simulink model "Comm_vec1111"  (R2018b)
settings: Solver=VariableStepAuto  StartTime=0.0  StopTime=4  MaxStep=1/(100*fn)  RelTol=1e-3
values from neighbouring files (symbols this model uses):
  A = sqrt(2/3)*[1 -0.5 -0.5; 0 sqrt(3)/2 -sqrt(3)/2; sqrt(0.5) sqrt(0.5) sqrt(0.5)]    [Comm_Vect.m]    (also in clarke_conc.m)
  Ai = inv(A)    [Comm_Vect.m]    (also in clarke_conc.m)
  fv = 0.0033    [Comm_Vect.m]    (also in clarke_conc.m)
  J = 0.05    [Comm_Vect.m]    (also in clarke_conc.m)
  Kond = 178    [Comm_Vect.m]
  Kpd = Rs/Kond    (= 0.0589887640449)    [Comm_Vect.m]
  Kpq = Rs/Kond    (= 0.0589887640449)    [Comm_Vect.m]
  Kpv = 1/Kond    (= 0.00561797752809)    [Comm_Vect.m]
  Ld = 0.245    [Comm_Vect.m]    (also in clarke_conc.m)
  Lq = 0.245    [Comm_Vect.m]    (also in clarke_conc.m)
  p = 60*fn/Nn    (= 2)    [Comm_Vect.m]    (also in clarke_conc.m)
  phi_f = 0.711    [Comm_Vect.m]    (also in clarke_conc.m)
  Rs = 10.5    [Comm_Vect.m]    (also in clarke_conc.m)
  Tid = Ld/Rs    (= 0.0233333333333)    [Comm_Vect.m]
  Tiq = Lq/Rs    (= 0.0233333333333)    [Comm_Vect.m]
  Tiv = J/fv    (= 15.1515151515)    [Comm_Vect.m]
  ws = 2*pi*fn/p    (= 157.079632679)    [Comm_Vect.m]    (also in clarke_conc.m)
undefined symbols (not defined in the file or in its folder): jsin
settings Model: Creator=cindyiskandar  LastModifiedBy=cindyiskandar

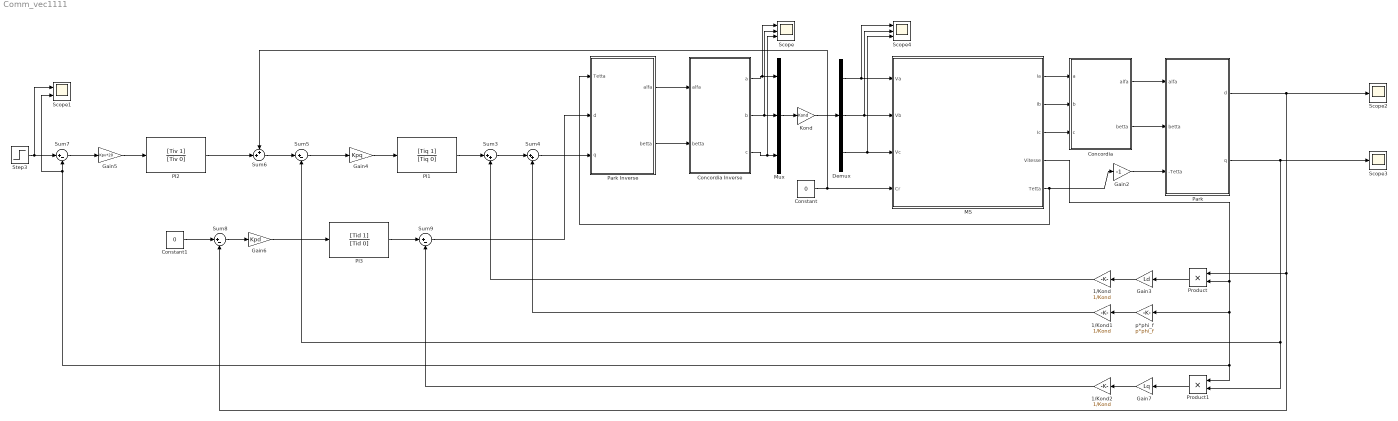
== system Comm_vec1111 ==
  1/Kond : Gain  Gain=1/Kond
  1/Kond1 : Gain  Gain=1/Kond
  1/Kond2 : Gain  Gain=1/Kond
  "Concordia " : Subsystem
  "Concordia Inverse " : Subsystem
  Constant : Constant  Value=0
  Constant1 : Constant  Value=0
  Demux : Demux  Outputs=3
  Gain2 : Gain  Gain=-1
  Gain3 : Gain  Gain=Ld
  Gain4 : Gain  Gain=Kpq
  Gain5 : Gain  Gain=Kpv*20
  Gain6 : Gain  Gain=Kpd
  Gain7 : Gain  Gain=Lq
  Kond : Gain  Gain=Kond
  MS : Subsystem
  Mux : Mux  Inputs=3
  PI1 : TransferFcn  Numerator=[Tiq 1]  Denominator=[Tiq 0]
  PI2 : TransferFcn  Numerator=[Tiv 1]  Denominator=[Tiv 0]
  PI3 : TransferFcn  Numerator=[Tid 1]  Denominator=[Tid 0]
  Park : Subsystem
  Park Inverse : Subsystem
  Product : Product
  Product1 : Product
  Scope : Scope  NumInputPorts=3
  Scope1 : Scope  NumInputPorts=2
  Scope2 : Scope
  Scope3 : Scope
  Scope4 : Scope  NumInputPorts=3
  Step3 : Step  Time=0  After=ws  SampleTime=0
  Sum3 : Sum  Inputs=|++
  Sum4 : Sum  Inputs=|++
  Sum{5,7..9} (4 alike) : Sum  Inputs=|+-
  Sum6 : Sum  Inputs=++|
  "p*phi_f " : Gain  Gain=p*phi_f
  wires:
  Park Inverse/2(betta) -> "Concordia Inverse "/2(betta)
  Step3/1 -> Scope1/1, Sum7/1
  "Concordia "/2("betta ") -> Park/2("betta ")
  Sum3/1 -> Sum4/1
  1/Kond2/1 -> Sum9/2
  "p*phi_f "/1 -> 1/Kond1/1
  Product/1 -> Gain3/1
  Gain5/1 -> PI2/1
  Constant1/1 -> Sum8/1
  Park/1(d) -> Scope2/1, Product/1, Sum8/2
  "Concordia Inverse "/2(b) -> Scope/2, Mux/2
  1/Kond1/1 -> Sum4/2
  PI1/1 -> Sum3/1
  Product1/1 -> Gain7/1
  Sum7/1 -> Gain5/1
  MS/5("Tetta ") -> Gain2/1, Park Inverse/1("Tetta ")
  Sum8/1 -> Gain6/1
  Park Inverse/1(alfa) -> "Concordia Inverse "/1(alfa)
  Gain7/1 -> 1/Kond2/1
  Mux/1 -> Kond/1
  "Concordia Inverse "/1(a) -> Scope/1, Mux/1
  Gain2/1 -> Park/3(-Tetta)
  MS/4(Vitesse) -> "p*phi_f "/1, Product1/1, Scope1/2, Sum7/2, Product/2
  Sum5/1 -> Gain4/1
  MS/3(Ic) -> "Concordia "/3(c)
  MS/2(Ib) -> "Concordia "/2("b ")
  Sum9/1 -> Park Inverse/2(d)
  Gain3/1 -> 1/Kond/1
  Gain6/1 -> PI3/1
  1/Kond/1 -> Sum3/2
  "Concordia "/1(alfa) -> Park/1(alfa)
  Gain4/1 -> PI1/1
  PI3/1 -> Sum9/1
  MS/1(Ia) -> "Concordia "/1("a ")
  Constant/1 -> MS/4(Cr), Sum6/1
  PI2/1 -> Sum6/2
  Sum4/1 -> Park Inverse/3("q ")
  Kond/1 -> Demux/1
  Park/2(q) -> Scope3/1, Product1/2, Sum5/2
  "Concordia Inverse "/3(c) -> Scope/3, Mux/3
  Demux/3 -> Scope4/3, MS/3(Vc)
  Demux/1 -> Scope4/1, MS/1(Va)
  Demux/2 -> MS/2(Vb), Scope4/2
  Sum6/1 -> Sum5/1

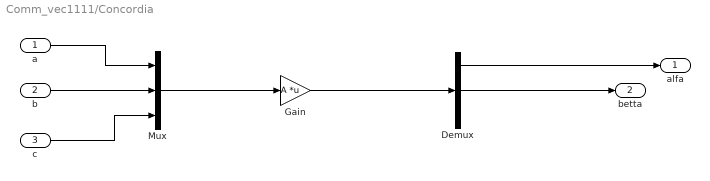
== system Comm_vec1111/Concordia  ==
  "a " : Inport
  "b " : Inport  Port=2
  c : Inport  Port=3
  Demux : Demux  Outputs=3
  Gain : Gain  Gain=A  Multiplication=Matrix(K*u) (u vector)
  Mux : Mux  Inputs=3
  alfa : Outport
  "betta " : Outport  Port=2
  wires:
  Demux/1 -> alfa/1
  "a "/1 -> Mux/1
  Mux/1 -> Gain/1
  Gain/1 -> Demux/1
  "b "/1 -> Mux/2
  c/1 -> Mux/3
  Demux/2 -> "betta "/1

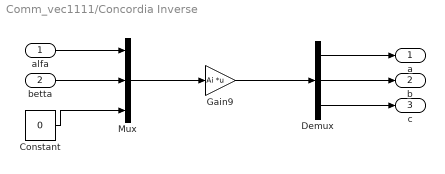
== system Comm_vec1111/Concordia Inverse  ==
  alfa : Inport
  betta : Inport  Port=2
  Constant : Constant  Value=0
  Demux : Demux  Outputs=3
  Gain9 : Gain  Gain=Ai  Multiplication=Matrix(K*u) (u vector)
  Mux : Mux  Inputs=3
  a : Outport
  b : Outport  Port=2
  c : Outport  Port=3
  wires:
  Demux/3 -> c/1
  Gain9/1 -> Demux/1
  Demux/1 -> a/1
  Demux/2 -> b/1
  betta/1 -> Mux/2
  alfa/1 -> Mux/1
  Mux/1 -> Gain9/1
  Constant/1 -> Mux/3

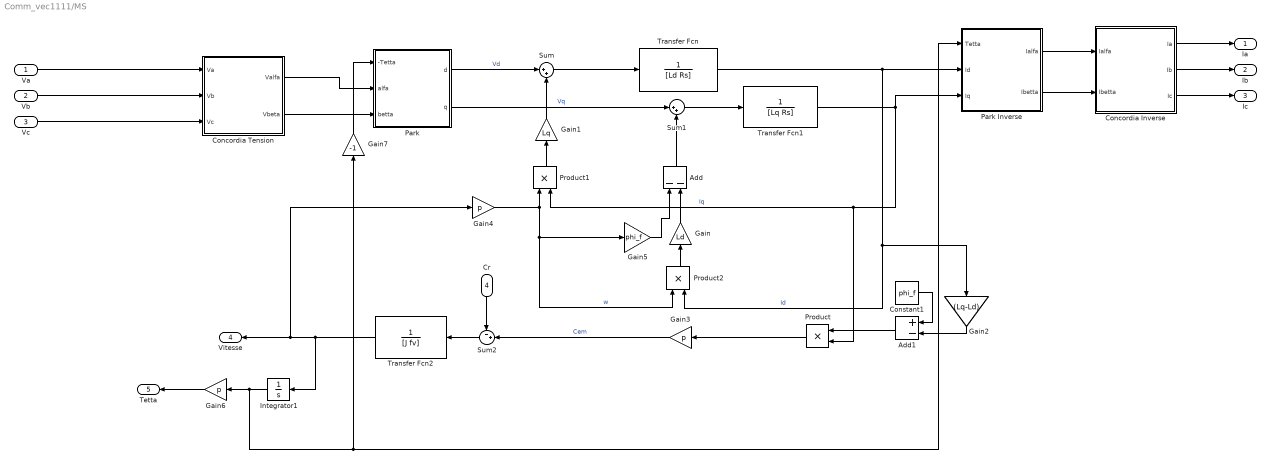
== system Comm_vec1111/MS ==
  Va : Inport
  Vb : Inport  Port=2
  Vc : Inport  Port=3
  Cr : Inport  Port=4
  Add : Sum  Inputs=--
  Add1 : Sum  Inputs=+-
  "Concordia Tension " : Subsystem
  "Concordia Inverse " : Subsystem
  Constant1 : Constant  Value=phi_f
  Gain : Gain  Gain=Ld
  Gain1 : Gain  Gain=Lq
  Gain2 : Gain  Gain=(Lq-Ld)
  Gain3 : Gain  Gain=p
  Gain4 : Gain  Gain=p
  Gain5 : Gain  Gain=phi_f
  Gain6 : Gain  Gain=p
  Gain7 : Gain  Gain=-1
  Integrator1 : Integrator  InitialCondition=ws
  Park : Subsystem
  Park Inverse : Subsystem
  Product : Product
  Product1 : Product
  Product2 : Product
  Sum : Sum  Inputs=|++
  Sum1 : Sum  Inputs=|++
  Sum2 : Sum  Inputs=-+|
  Transfer Fcn : TransferFcn  Denominator=[Ld Rs]
  Transfer Fcn1 : TransferFcn  Denominator=[Lq Rs]
  Transfer Fcn2 : TransferFcn  Denominator=[J fv]
  Ia : Outport
  Ib : Outport  Port=2
  Ic : Outport  Port=3
  Vitesse : Outport  Port=4
  "Tetta " : Outport  Port=5
  wires:
  Gain2/1 -> Add1/2
  Sum1/1 -> Transfer Fcn1/1
  Gain1/1 -> Sum/2
  Va/1 -> "Concordia Tension "/1("Va ")
  Gain/1 -> Add/2
  "Concordia Inverse "/2(Ib) -> Ib/1
  Vb/1 -> "Concordia Tension "/2("Vb ")
  Constant1/1 -> Add1/1
  Transfer Fcn1/1 -> Park Inverse/3("Iq "), Product1/2, Product/2  "Iq"
  "Concordia Inverse "/3(Ic) -> Ic/1
  Add1/1 -> Product/1
  Add/1 -> Sum1/2
  Park Inverse/2(Ibetta) -> "Concordia Inverse "/2(Ibetta)
  Park Inverse/1(Ialfa) -> "Concordia Inverse "/1(Ialfa)
  Sum/1 -> Transfer Fcn/1
  "Concordia Tension "/2("Vbeta ") -> Park/3("betta ")
  "Concordia Tension "/1(Valfa) -> Park/2(alfa)
  Vc/1 -> "Concordia Tension "/3(Vc)
  "Concordia Inverse "/1(Ia) -> Ia/1
  Park/1(d) -> Sum/1  "Vd"
  Transfer Fcn/1 -> Product2/2, Gain2/1, Park Inverse/2(Id)  "Id"
  Park/2(q) -> Sum1/1  "Vq"
  Product/1 -> Gain3/1
  Cr/1 -> Sum2/1
  Sum2/1 -> Transfer Fcn2/1
  Transfer Fcn2/1 -> Gain4/1, Vitesse/1, Integrator1/1
  Product1/1 -> Gain1/1
  Gain4/1 -> Product2/1, Gain5/1, Product1/1  "w"
  Product2/1 -> Gain/1
  Gain5/1 -> Add/1
  Gain6/1 -> "Tetta "/1
  Integrator1/1 -> Gain7/1, Park Inverse/1("Tetta "), Gain6/1
  Gain7/1 -> Park/1(-Tetta)
  Gain3/1 -> Sum2/2  "Cem"

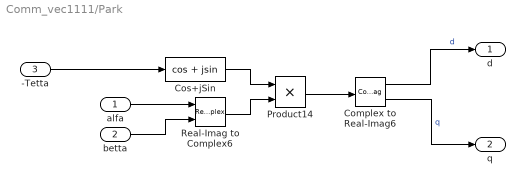
== system Comm_vec1111/Park ==
  alfa : Inport
  "betta " : Inport  Port=2
  -Tetta : Inport  Port=3
  Complex to Real-Imag6 : ComplexToRealImag
  Cos+jSin : Trigonometry  Operator=cos + jsin
  Product14 : Product
  Real-Imag to Complex6 : RealImagToComplex
  d : Outport
  q : Outport  Port=2
  wires:
  alfa/1 -> Real-Imag to Complex6/1
  Product14/1 -> Complex to Real-Imag6/1
  "betta "/1 -> Real-Imag to Complex6/2
  Complex to Real-Imag6/1 -> d/1  "d"
  Complex to Real-Imag6/2 -> q/1  "q"
  Real-Imag to Complex6/1 -> Product14/2
  Cos+jSin/1 -> Product14/1
  -Tetta/1 -> Cos+jSin/1

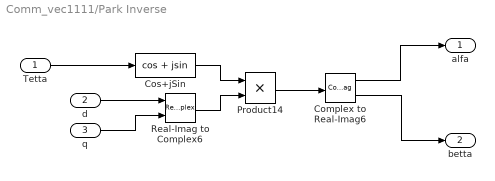
== system Comm_vec1111/Park Inverse ==
  "Tetta " : Inport
  d : Inport  Port=2
  "q " : Inport  Port=3
  Complex to Real-Imag6 : ComplexToRealImag
  Cos+jSin : Trigonometry  Operator=cos + jsin
  Product14 : Product
  Real-Imag to Complex6 : RealImagToComplex
  alfa : Outport
  betta : Outport  Port=2
  wires:
  d/1 -> Real-Imag to Complex6/1
  Product14/1 -> Complex to Real-Imag6/1
  "q "/1 -> Real-Imag to Complex6/2
  Complex to Real-Imag6/1 -> alfa/1
  Complex to Real-Imag6/2 -> betta/1
  Real-Imag to Complex6/1 -> Product14/2
  Cos+jSin/1 -> Product14/1
  "Tetta "/1 -> Cos+jSin/1

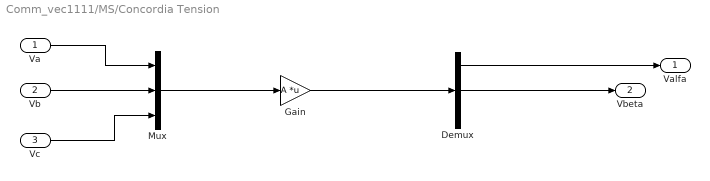
== system Comm_vec1111/MS/Concordia Tension  ==
  "Va " : Inport
  "Vb " : Inport  Port=2
  Vc : Inport  Port=3
  Demux : Demux  Outputs=3
  Gain : Gain  Gain=A  Multiplication=Matrix(K*u) (u vector)
  Mux : Mux  Inputs=3
  Valfa : Outport
  "Vbeta " : Outport  Port=2
  wires:
  Demux/1 -> Valfa/1
  "Va "/1 -> Mux/1
  Mux/1 -> Gain/1
  Gain/1 -> Demux/1
  "Vb "/1 -> Mux/2
  Vc/1 -> Mux/3
  Demux/2 -> "Vbeta "/1

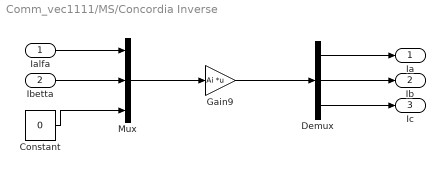
== system Comm_vec1111/MS/Concordia Inverse  ==
  Ialfa : Inport
  Ibetta : Inport  Port=2
  Constant : Constant  Value=0
  Demux : Demux  Outputs=3
  Gain9 : Gain  Gain=Ai  Multiplication=Matrix(K*u) (u vector)
  Mux : Mux  Inputs=3
  Ia : Outport
  Ib : Outport  Port=2
  Ic : Outport  Port=3
  wires:
  Demux/3 -> Ic/1
  Gain9/1 -> Demux/1
  Demux/1 -> Ia/1
  Demux/2 -> Ib/1
  Ibetta/1 -> Mux/2
  Ialfa/1 -> Mux/1
  Mux/1 -> Gain9/1
  Constant/1 -> Mux/3

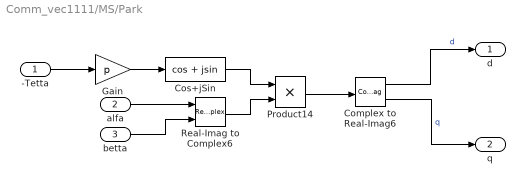
== system Comm_vec1111/MS/Park ==
  -Tetta : Inport
  alfa : Inport  Port=2
  "betta " : Inport  Port=3
  Complex to Real-Imag6 : ComplexToRealImag
  Cos+jSin : Trigonometry  Operator=cos + jsin
  Gain : Gain  Gain=p
  Product14 : Product
  Real-Imag to Complex6 : RealImagToComplex
  d : Outport
  q : Outport  Port=2
  wires:
  alfa/1 -> Real-Imag to Complex6/1
  Product14/1 -> Complex to Real-Imag6/1
  "betta "/1 -> Real-Imag to Complex6/2
  Complex to Real-Imag6/1 -> d/1  "d"
  Complex to Real-Imag6/2 -> q/1  "q"
  Real-Imag to Complex6/1 -> Product14/2
  Cos+jSin/1 -> Product14/1
  Gain/1 -> Cos+jSin/1
  -Tetta/1 -> Gain/1

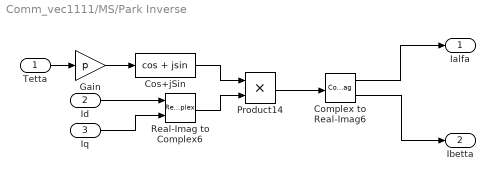
== system Comm_vec1111/MS/Park Inverse ==
  "Tetta " : Inport
  Id : Inport  Port=2
  "Iq " : Inport  Port=3
  Complex to Real-Imag6 : ComplexToRealImag
  Cos+jSin : Trigonometry  Operator=cos + jsin
  Gain : Gain  Gain=p
  Product14 : Product
  Real-Imag to Complex6 : RealImagToComplex
  Ialfa : Outport
  Ibetta : Outport  Port=2
  wires:
  Id/1 -> Real-Imag to Complex6/1
  Product14/1 -> Complex to Real-Imag6/1
  "Iq "/1 -> Real-Imag to Complex6/2
  Complex to Real-Imag6/1 -> Ialfa/1
  Complex to Real-Imag6/2 -> Ibetta/1
  Real-Imag to Complex6/1 -> Product14/2
  Cos+jSin/1 -> Product14/1
  Gain/1 -> Cos+jSin/1
  "Tetta "/1 -> Gain/1
